simulink model "Modelo_Entrenamiento"  (R2025b)
settings: Solver=VariableStepAuto  StartTime=0.0  StopTime=5000  RelTol=1e-3
libraries: spsGroundLib x2, spsParallelRLCBranchLib x2, spsControlledVoltageSourceLib x1, spsCurrentMeasurementLib x1, spsVariableResistorLib x1, spsVoltageMeasurementLib x1, spspowerguiLib x1
settings Model: Creator=Hp  LastModifiedBy=joseA

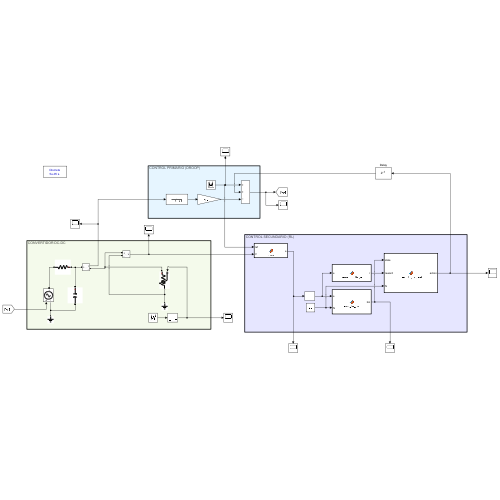
[thumbnail: Simulink's stored preview of the top-level diagram]
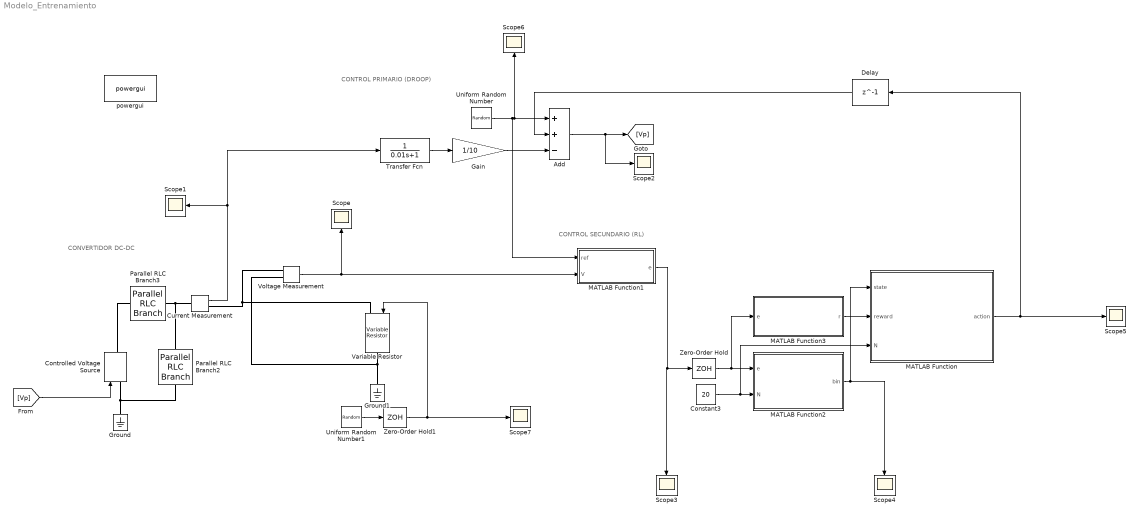
== system Modelo_Entrenamiento ==
  note: CONVERTIDOR DC-DC
  note: CONTROL PRIMARIO (DROOP)
  note: CONTROL SECUNDARIO (RL)
  Add : Sum  Inputs=++-
  Constant3 : Constant  Value=20
  Controlled Voltage Source : spsControlledVoltageSourceLib/Controlled Voltage Source  Initialize=on  Source_Type=DC  Amplitude=0  Phase=0  Frequency=0  Measurements=None
  Current Measurement : spsCurrentMeasurementLib/Current Measurement  PhasorSimulation=off  OutputType=Complex  PSBequivalent=0
  Delay : Delay  DelayLength=1  InitialCondition=0  UseCircularBuffer=on
  Gain : Gain  Gain=1/10
  Ground : spsGroundLib/Ground  LConnTagsString=a
  Ground1 : spsGroundLib/Ground  LConnTagsString=a
  MATLAB Function : MATLAB Function  TreatAsAtomicUnit=on
  MATLAB Function1 : MATLAB Function  TreatAsAtomicUnit=on
  MATLAB Function2 : MATLAB Function  TreatAsAtomicUnit=on
  MATLAB Function3 : MATLAB Function  TreatAsAtomicUnit=on
  Parallel RLC Branch2 : spsParallelRLCBranchLib/Parallel RLC Branch  LConnTagsString=a  RConnTagsString=__new0  BranchType=C  Resistance=2  Inductance=1e-3  SetiL0=off  InitialCurrent=0  Capacitance=1e-6  Setx0=off  InitialVoltage=Vc0  Measurements=None
  Parallel RLC Branch3 : spsParallelRLCBranchLib/Parallel RLC Branch  LConnTagsString=a  RConnTagsString=__new0  BranchType=R  Resistance=0.01  Inductance=1e-3  SetiL0=off  InitialCurrent=0  Capacitance=1e-6  Setx0=off  InitialVoltage=0  Measurements=None
  Scope{,1..7} (8 alike) : Scope
      Scope settings: ActiveDisplayYMinimum=-20.33002  ActiveDisplayYMaximum=29.97059
      Scope1 settings: ActiveDisplayYMinimum=-0.70648  ActiveDisplayYMaximum=6.35828
      Scope2 settings: ActiveDisplayYMinimum=-20.47791  ActiveDisplayYMaximum=30.08142  DataLoggingVariableName=ScopeData2
      Scope3 settings: ActiveDisplayYMinimum=-5571.34515  ActiveDisplayYMaximum=2895.1214  DataLoggingVariableName=ScopeData3
      Scope4 settings: ActiveDisplayYMinimum=-1.375  ActiveDisplayYMaximum=22.375
      Scope5 settings: ActiveDisplayYMinimum=-6.25  ActiveDisplayYMaximum=6.25
      Scope6 settings: ActiveDisplayYMinimum=-13.74987  ActiveDisplayYMaximum=23.74998  DataLoggingVariableName=ScopeData2
      Scope7 settings: ActiveDisplayYMinimum=-0.10249  ActiveDisplayYMaximum=11.10803  DataLoggingVariableName=ScopeData3
  Transfer Fcn : TransferFcn  Denominator=[0.01 1]
  Uniform Random Number : UniformRandomNumber  Minimum=-10  Maximum=20  Seed=0.5  SampleTime=0.1
  Uniform Random Number1 : UniformRandomNumber  Minimum=1  Maximum=10  Seed=0.5  SampleTime=0.1
  Variable Resistor : spsVariableResistorLib/Variable Resistor  Rabsmin=1e-3
      settings: LibrarySourceBlock=sps_lib/Passives/Variable Resistor
  Voltage Measurement : spsVoltageMeasurementLib/Voltage Measurement  PhasorSimulation=off  OutputType=Complex  PSBequivalent=0
  Zero-Order Hold : ZeroOrderHold  SampleTime=0.1
  Zero-Order Hold1 : ZeroOrderHold  SampleTime=5
  powergui : spspowerguiLib/powergui  Priority=1  SimulationMode=Discrete  SampleTime=50e-6  frequency=60  Iterations=50  frequencyindice=0  Pbase=100e6  ErrMax=1e-4  UnitsV=kV  UnitsW=MW  buscounter=0  FunctionMessages=off  echomessages=off  EnableUseOfTLC=off  CurrentSourceSwitches=off  DisableSnubberDevices=off  DisableRonSwitches=off  DisableVfSwitches=off  DisplayEquations=off  AutomaticDiscreteSolvers=off  SolverType=Tustin/Backward Euler (TBE)  Interpol=off  ExternalGateDelay=off  methode=off  Ts=100  x0status=blocks  SPID=on  SwTol=0  HookPort=off  NonlinearTolerance=1e-4  nMaxIteration=100  ContinueOnMaxIteration=off  RestoreLinks=warning  ResistiveCurrentMeasurement=off  Frange=[0:2:500]  Ylog=off  Xlog=on  ShowGrid=off  save=off  variable=ZData  structure=0  ZoomFFT=off  StartTime=0.0  cycles=1  DisplayStyle=1  fundamental=60  FreqAxis=off  MaxFrequency=1000  frequencyindicesteady=1  RmsSteady=1  display=off
  wires:
  Current Measurement/1 -> Transfer Fcn/1, Scope1/1
  Add/1 -> Scope2/1, [Vp]
  Transfer Fcn/1 -> Gain/1
  MATLAB Function1/1(e) -> Zero-Order Hold/1, Scope3/1
  Zero-Order Hold/1 -> MATLAB Function3/1(e), MATLAB Function2/1(e)
  [Vp] -> Controlled Voltage Source/1
  Voltage Measurement/1 -> Scope/1, MATLAB Function1/2(V)
  Uniform Random Number/1 -> Add/1, Scope6/1, MATLAB Function1/1(ref)
  Constant3/1 -> MATLAB Function/3(N), MATLAB Function2/2(N)
  MATLAB Function3/1(r) -> MATLAB Function/2(reward)
  MATLAB Function2/1(bin) -> MATLAB Function/1(state), Scope4/1
  MATLAB Function/1(action) -> Delay/1, Scope5/1
  Uniform Random Number1/1 -> Zero-Order Hold1/1
  Zero-Order Hold1/1 -> Scope7/1, Variable Resistor/1
  Gain/1 -> Add/3
  Delay/1 -> Add/2
  connections:
  Current Measurement/RConn1 -- Voltage Measurement/LConn1 -- Variable Resistor/LConn1
  Ground/LConn1 -- Controlled Voltage Source/LConn1 -- Parallel RLC Branch2/RConn1
  Ground1/LConn1 -- Variable Resistor/RConn1 -- Voltage Measurement/LConn2
  Current Measurement/LConn1 -- Parallel RLC Branch2/LConn1 -- Parallel RLC Branch3/LConn1
  Controlled Voltage Source/RConn1 -- Parallel RLC Branch3/RConn1

== matlab function Modelo_Entrenamiento/MATLAB Function1 ==
  data: ref input; e output; V input
function e = error(ref,V)


e=(ref-V)/ref;

end

== matlab function Modelo_Entrenamiento/MATLAB Function ==
  data: state input; action output; reward input; N input
function action = qlearning_agent(state, reward, N)

persistent Q epsilon alpha gamma lastState lastAction isFirstCall

% ----- Acciones discretas -----
actions = -5:0.1:5;
A = numel(actions); % tamaño de actions

% ----- Inicialización -----
if isempty(Q)
    Q = zeros(N, A);
    epsilon = 0.8;
    epsilonMin  = 0.05;
    epsilonDecay = 0.995;
    epsilon = max(epsilonMin, epsilon * epsilonDecay);
    alpha   = 0.1;
    gamma   = 0.9;


    lastState  = state;
    lastAction = 0;
    isFirstCall = true;
end

% ----- Saturar estado -----
%state = max(1, min(N, round(state)));

% ----- Actualización Q -----
if ~isFirstCall
    s_prev = lastState;
    a_prev = lastAction;

    maxQ = max(Q(state, :));

    Q(s_prev, a_prev) = Q(s_prev, a_prev) + ...
        alpha * (reward + gamma * maxQ - Q(s_prev, a_prev));

    assignin('base','Q_table',Q);
end

% ----- Política epsilon-greedy -----
if rand < epsilon
    actionIdx = randi(A);            % explorar
else
    [~, actionIdx] = max(Q(state,:));% explotar
end

% ----- Salida -----
action = actions(actionIdx);

% ----- Guardar para siguiente paso -----
lastState  = state;
lastAction = actionIdx;
isFirstCall = false;

end

== matlab function Modelo_Entrenamiento/MATLAB Function2 ==
  data: e input; bin output; N input
function bin = error_to_bin(e,N)

error_min = -2;
error_max =  2;

error_edges = linspace(error_min, error_max, N+1);


bin = discretize(e, error_edges);

% Protección contra NaN
if isnan(bin)
    if e < error_edges(1)
        bin = 1;
    else
        bin = N;
    end
end

== matlab function Modelo_Entrenamiento/MATLAB Function3 ==
  data: e input; r output
function r = reward_voltage(e)


r = - (2*e)^2;

end
